simulink model "SSC_EigvalPlacement"  (R2024b)
settings: Solver=VariableStepAuto  StartTime=0.0  StopTime=10.0  RelTol=1e-3
undefined symbols (not defined in the file or in its folder): drv, Nu, Nx, rpm2rads, ssc
settings Model: Creator=llp  LastModifiedBy=fede

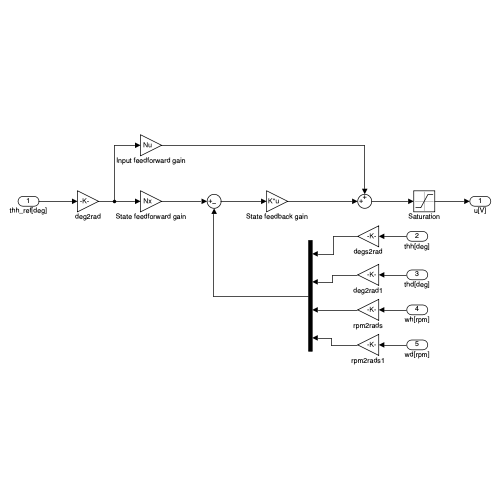
[thumbnail: Simulink's stored preview of the top-level diagram]
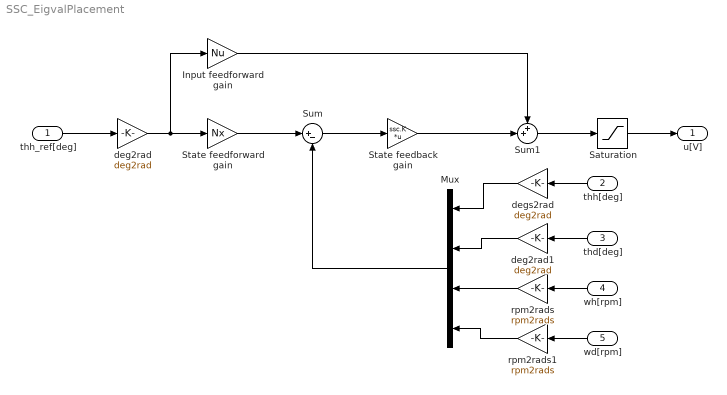
== system SSC_EigvalPlacement ==
  thh_ref[deg] : Inport
  thh[deg] : Inport  Port=2
  thd[deg] : Inport  Port=3
  wh[rpm] : Inport  Port=4
  wd[rpm] : Inport  Port=5
  Input feedforward gain : Gain  Gain=Nu
  Mux : Mux
  Saturation : Saturate  UpperLimit=drv.outmax  LowerLimit=-drv.outmax
  State feedback gain : Gain  Gain=ssc.K  Multiplication=Matrix(K*u)
  State feedforward gain : Gain  Gain=Nx
  Sum : Sum  Inputs=|+-
  Sum1 : Sum  Inputs=++|
  deg2rad : Gain  Gain=deg2rad
  deg2rad1 : Gain  Gain=deg2rad
  degs2rad : Gain  Gain=deg2rad
  rpm2rads : Gain  Gain=rpm2rads
  rpm2rads1 : Gain  Gain=rpm2rads
  u[V] : Outport
  wires:
  Sum/1 -> State feedback gain/1
  Mux/1 -> Sum/2
  thd[deg]/1 -> deg2rad1/1
  deg2rad1/1 -> Mux/2
  State feedback gain/1 -> Sum1/2
  deg2rad/1 -> Input feedforward gain/1, State feedforward gain/1
  Saturation/1 -> u[V]/1
  thh_ref[deg]/1 -> deg2rad/1
  Sum1/1 -> Saturation/1
  Input feedforward gain/1 -> Sum1/1
  State feedforward gain/1 -> Sum/1
  degs2rad/1 -> Mux/1
  thh[deg]/1 -> degs2rad/1
  wh[rpm]/1 -> rpm2rads/1
  wd[rpm]/1 -> rpm2rads1/1
  rpm2rads/1 -> Mux/3
  rpm2rads1/1 -> Mux/4
